simulink model "Project3"  (R2024a)
settings: Solver=VariableStepAuto  StartTime=0.0  StopTime=10.0  MaxStep=0.05  RelTol=1e-3
values from neighbouring files (symbols this model uses):
  b = 3.5077E-6    (= 3.5077e-06)    [Project10Mscript.m]    (also in Project3Mscript.m = 2; Project4Mscript.m = 0; Project7Mscript.m = 10)
  F = 1    [Project3Mscript.m]    (also in Project4Mscript.m; Project7Mscript.m; Project_2Mscript.m = 5)
  k = 20    [Project3Mscript.m]    (also in Project4Mscript.m; Project7Mscript.m)
  Kd = 1000    [Project10Mscript.m]    (also in Project6Mscript.m = 3; Project7Mscript.m = 500)
  Ki = 50    [Project10Mscript.m]    (also in Project6Mscript.m = 1; Project7Mscript.m)
  Kp = 500    [Project10Mscript.m]    (also in Project6Mscript.m = 2; Project7Mscript.m = 350)
  M = 1    [Project3Mscript.m]    (also in Project4Mscript.m; Project7Mscript.m)
settings Model: Creator=harsh  LastModifiedBy=harsh

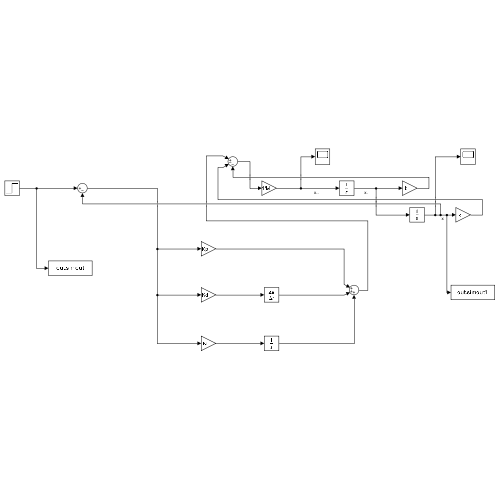
[thumbnail: Simulink's stored preview of the top-level diagram]
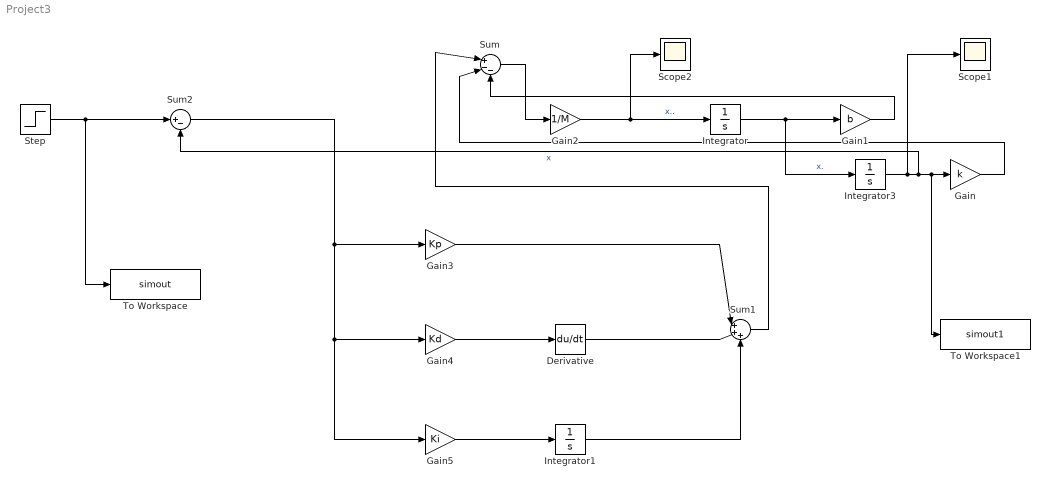
== system Project3 ==
  Derivative : Derivative
  Gain : Gain  Gain=k
  Gain1 : Gain  Gain=b
  Gain2 : Gain  Gain=1/M
  Gain3 : Gain  Gain=Kp
  Gain4 : Gain  Gain=Kd
  Gain5 : Gain  Gain=Ki
  Integrator : Integrator
  Integrator1 : Integrator
  Integrator3 : Integrator
  Scope1 : Scope
  Scope2 : Scope
  Step : Step  After=F  SampleTime=0
  Sum : Sum  Inputs=|+--
  Sum1 : Sum  Inputs=|+++
  Sum2 : Sum  Inputs=|+-
  To Workspace : ToWorkspace  VariableName=simout  SaveFormat=Timeseries  SampleTime=-1
  To Workspace1 : ToWorkspace  VariableName=simout1  SaveFormat=Timeseries  SampleTime=-1
  wires:
  Integrator/1 -> Integrator3/1, Gain1/1  "x."
  Gain2/1 -> Scope2/1, Integrator/1  "x.."
  Gain1/1 -> Sum/3
  Integrator3/1 -> Scope1/1, To Workspace1/1, Gain/1, Sum2/2  "x"
  Gain/1 -> Sum/2
  Sum/1 -> Gain2/1
  Gain4/1 -> Derivative/1
  Sum2/1 -> Gain5/1, Gain4/1, Gain3/1
  Integrator1/1 -> Sum1/3
  Gain5/1 -> Integrator1/1
  Derivative/1 -> Sum1/2
  Gain3/1 -> Sum1/1
  Sum1/1 -> Sum/1
  Step/1 -> To Workspace/1, Sum2/1
